simulink model "SF020A_HwAgTrakgServo"  (R2013b)
settings: Solver=FixedStepDiscrete  SolverMode=SingleTasking  StartTime=0.0  StopTime=1  FixedStep=0.002  RelTol=1e-3
undefined symbols (not defined in the file): ARCHGLBPRM_2MILLISEC_SEC_F32, HwAgTrakgServoEnaRate, HwAgTrakgServoExecRate, HwAgTrakgServoMaxRamp, HwAgTrakgServoPidLim, HwAgTrakgServoRampCmpl, SYSGLBPRM_MOTTQCMDHILIM_MOTNWTMTR_F32, SYSGLBPRM_MOTTQCMDLOLIM_MOTNWTMTR_F32
libraries: FixdToFloat x9, FloatToFixd x8, LnrIntrpn x7, NxtrLim x7, Fil x6, simulink x3, NxtrAbslt x2, BilnrIntrpnCmnX x2, NxtrSign x2
(part 2 of 2)

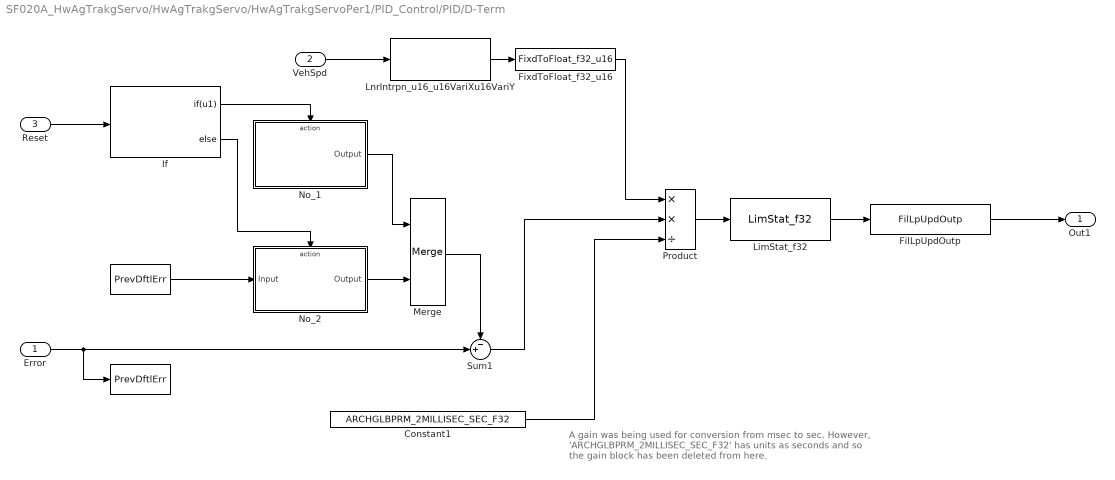
== system SF020A_HwAgTrakgServo/HwAgTrakgServo/HwAgTrakgServoPer1/PID_Control/PID/D-Term ==
  note: A gain was being used for conversion from msec to sec.
      | However, 'ARCHGLBPRM_2MILLISEC_SEC_F32' has units
      | as seconds and so the gain block has been deleted from here.
  Error : Inport
  VehSpd : Inport  RequirementInfo={'linktype_rmi_doors' '0000a533 (/E-STEER Core/SubSystem Specifications/Application Functions/SF020A Position Tracking Servo)' '#SF020A_120' 'true' 'REQ:SF020A_120' '' } %GIDa_d32483ba_765c_4e7c_9854_4c9d7c34dac7  Port=2
  Reset : Inport  Port=3
  "  " : DataStoreWrite  RequirementInfo={'linktype_rmi_doors' '0000a533 (/E-STEER Core/SubSystem Specifications/Application Functions/SF020A Position Tracking Servo)' '#SF020A_120' 'true' 'REQ:SF020A_120' '' } %GIDa_7a2ff437_0271_4ce9_818a_ade8654f46bb  DataStoreName=PrevDftlErr
  " " : DataStoreRead  RequirementInfo={'linktype_rmi_doors' '0000a533 (/E-STEER Core/SubSystem Specifications/Application Functions/SF020A Position Tracking Servo)' '#SF020A_121' 'true' 'REQ:SF020A_121' '' } %GIDa_b646c468_9863_49bd_b902_8e22191691a8  DataStoreName=PrevDftlErr
  Constant1 : Constant  RequirementInfo={'linktype_rmi_doors' '0000a533 (/E-STEER Core/SubSystem Specifications/Application Functions/SF020A Position Tracking Servo)' '#SF020A_120' 'true' 'REQ:SF020A_120' '' } %GIDa_1ecc393f_7cc1_4c4e_8080_3b7a410d844f  Value=ARCHGLBPRM_2MILLISEC_SEC_F32
  FilLpUpdOutp : Fil/FilLpUpdOutp  RequirementInfo="{'linktype_rmi_doors' '0000a533 (/E-STEER Core/SubSystem Specifications/Application Functions/SF020A Position Tracking Servo)' '#SF020A_120' 'true' 'REQ:  SF020A_120' '' } %GIDa_b8410d6a_59fe_4dcb_bcc7_9a13096b2737"  StVar=DftlTermLpFil
      settings: AttributesFormatString=StVar: %<StVar>
  FixdToFloat_f32_u16 : FixdToFloat/FixdToFloat_f32_u16  RequirementInfo="{'linktype_rmi_doors' '0000a533 (/E-STEER Core/SubSystem Specifications/Application Functions/SF020A Position Tracking Servo)' '#SF020A_120' 'true' 'REQ:  SF020A_120' '' } %GIDa_8cac592f_9679_46eb_895c_0d05cfe3ff7b"  Param1=16
  If : If  RequirementInfo={'linktype_rmi_doors' '0000a533 (/E-STEER Core/SubSystem Specifications/Application Functions/SF020A Position Tracking Servo)' '#SF020A_121' 'true' 'REQ:SF020A_121' '' } %GIDa_2482da2c_29e3_486b_be60_b311b38fc278  IfExpression=u1
  LimStat_f32 : NxtrLim/LimStat_f32  RequirementInfo="{'linktype_rmi_doors' '0000a533 (/E-STEER Core/SubSystem Specifications/Application Functions/SF020A Position Tracking Servo)' '#SF020A_120' 'true' 'REQ:  SF020A_120' '' } %GIDa_56604264_d76a_420a_89c8_0243c47d2796"  LoLim=DFTLTERMMIN_MOTNWTMTR_F32  HiLim=DFTLTERMMAX_MOTNWTMTR_F32
      settings: AttributesFormatString=|
      | Low Limit: %<LoLim>
      | High Limit:%<HiLim>
  LnrIntrpn_u16_u16VariXu16VariY : LnrIntrpn/LnrIntrpn_u16_u16VariXu16VariY  RequirementInfo="{'linktype_rmi_doors' '0000a533 (/E-STEER Core/SubSystem Specifications/Application Functions/SF020A Position Tracking Servo)' '#SF020A_120' 'true' 'REQ:  SF020A_120' '' ; 'linktype_rmi_doors' '0000a533 (/E-STEER Core/SubSystem Specifications/Application Functions/SF020A Position Tracking Servo)' '#SF020A_121' 'true' 'REQ:  SF020A_121' '' } %GIDa_2e6fa66c_d77a_4943_945e_e25c3e6f5b3b"  XTbl=HwAgTrakgServoVehSpdBasd  YTbl=HwAgTrakgServoDftlGainY
      settings: AttributesFormatString=Lnr ( u16VariX , u16VariY )
  Merge : Merge  RequirementInfo={'linktype_rmi_doors' '0000a533 (/E-STEER Core/SubSystem Specifications/Application Functions/SF020A Position Tracking Servo)' '#SF020A_121' 'true' 'REQ:SF020A_121' '' } %GIDa_db000ce9_21e4_46f6_81ad_8c041347f9e5
  No_1 : Subsystem  RequirementInfo={'linktype_rmi_doors' '0000a533 (/E-STEER Core/SubSystem Specifications/Application Functions/SF020A Position Tracking Servo)' '#SF020A_121' 'true' 'REQ:SF020A_121' '' } %GIDa_913a8a21_a22e_47bf_9e83_df1d046cce8d  TreatAsAtomicUnit=on
  No_2 : Subsystem  RequirementInfo={'linktype_rmi_doors' '0000a533 (/E-STEER Core/SubSystem Specifications/Application Functions/SF020A Position Tracking Servo)' '#SF020A_121' 'true' 'REQ:SF020A_121' '' } %GIDa_9df1ffb9_cc87_486c_93e5_5eb2c3c347a7  TreatAsAtomicUnit=on
  Product : Product  RequirementInfo={'linktype_rmi_doors' '0000a533 (/E-STEER Core/SubSystem Specifications/Application Functions/SF020A Position Tracking Servo)' '#SF020A_120' 'true' 'REQ:SF020A_120' '' } %GIDa_10f02c07_eab9_451a_9a4c_01a4745aac1a  Inputs=**/  RndMeth=Zero
  Sum1 : Sum  RequirementInfo={'linktype_rmi_doors' '0000a533 (/E-STEER Core/SubSystem Specifications/Application Functions/SF020A Position Tracking Servo)' '#SF020A_120' 'true' 'REQ:SF020A_120' '' } %GIDa_669423b0_1be1_4fee_ba39_26e793d23548  Inputs=-+|
  Out1 : Outport
  wires:
  Sum1/1 -> Product/2
  Product/1 -> LimStat_f32/1
  LimStat_f32/1 -> FilLpUpdOutp/1
  FilLpUpdOutp/1 -> Out1/1
  Constant1/1 -> Product/3
  VehSpd/1 -> LnrIntrpn_u16_u16VariXu16VariY/1
  LnrIntrpn_u16_u16VariXu16VariY/1 -> FixdToFloat_f32_u16/1
  FixdToFloat_f32_u16/1 -> Product/1
  If/1 -> No_1/Action
  No_1/1(Output) -> Merge/1
  Merge/1 -> Sum1/1
  If/2 -> No_2/Action
  No_2/1(Output) -> Merge/2
  Reset/1 -> If/1
  Error/1 -> "  "/1, Sum1/2
  " "/1 -> No_2/1(Input)

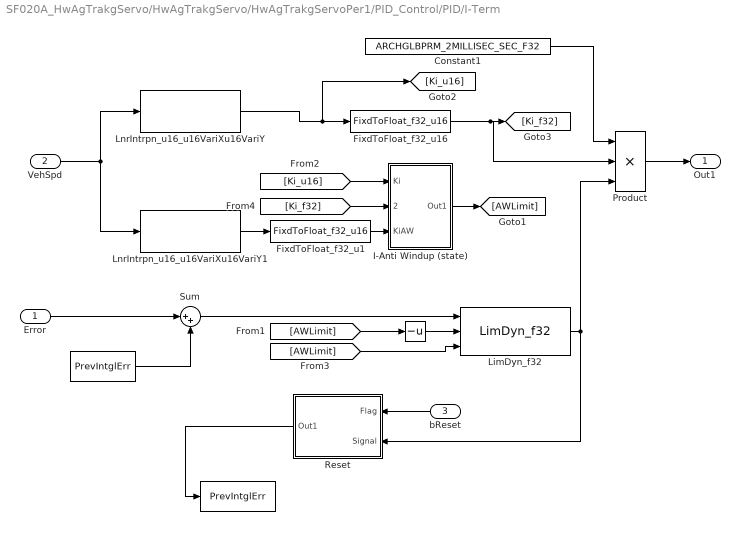
== system SF020A_HwAgTrakgServo/HwAgTrakgServo/HwAgTrakgServoPer1/PID_Control/PID/I-Term ==
  Error : Inport
  VehSpd : Inport  Port=2
  bReset : Inport  RequirementInfo={'linktype_rmi_doors' '0000a533 (/E-STEER Core/SubSystem Specifications/Application Functions/SF020A Position Tracking Servo)' '#SF020A_118' 'true' 'REQ:SF020A_118' '' } %GIDa_42cbd73d_d21d_4d14_befd_3c7d0ce0296a  Port=3
  " " : UnaryMinus  RequirementInfo={'linktype_rmi_doors' '0000a533 (/E-STEER Core/SubSystem Specifications/Application Functions/SF020A Position Tracking Servo)' '#SF020A_117' 'true' 'REQ:SF020A_117' '' } %GIDa_89f9ccfb_a876_46d8_9437_2574eb60ea80
  "    " : DataStoreRead  RequirementInfo={'linktype_rmi_doors' '0000a533 (/E-STEER Core/SubSystem Specifications/Application Functions/SF020A Position Tracking Servo)' '#SF020A_116' 'true' 'REQ:SF020A_116' '' } %GIDa_32ef5a5c_1147_48c1_a2b1_c99166101285  DataStoreName=PrevIntglErr
  "                      " : DataStoreWrite  RequirementInfo={'linktype_rmi_doors' '0000a533 (/E-STEER Core/SubSystem Specifications/Application Functions/SF020A Position Tracking Servo)' '#SF020A_118' 'true' 'REQ:SF020A_118' '' } %GIDa_fefcbefd_ce0f_4bfb_82a6_01cc1f5b96d1  DataStoreName=PrevIntglErr
  Constant1 : Constant  RequirementInfo={'linktype_rmi_doors' '0000a533 (/E-STEER Core/SubSystem Specifications/Application Functions/SF020A Position Tracking Servo)' '#SF020A_116' 'true' 'REQ:SF020A_116' '' } %GIDa_c7ba7a95_a44d_4b4f_9268_9abd4fc5ade3  Value=ARCHGLBPRM_2MILLISEC_SEC_F32
  FixdToFloat_f32_u1 : FixdToFloat/FixdToFloat_f32_u16  RequirementInfo="{'linktype_rmi_doors' '0000a533 (/E-STEER Core/SubSystem Specifications/Application Functions/SF020A Position Tracking Servo)' '#SF020A_117' 'true' 'REQ:  SF020A_117' '' } %GIDa_9607823e_5536_4c8d_af66_ea7d7950732e"  Param1=6
  FixdToFloat_f32_u16 : FixdToFloat/FixdToFloat_f32_u16  RequirementInfo="{'linktype_rmi_doors' '0000a533 (/E-STEER Core/SubSystem Specifications/Application Functions/SF020A Position Tracking Servo)' '#SF020A_116' 'true' 'REQ:  SF020A_116' '' } %GIDa_4b7f174a_bb9c_4a9b_b796_dd3c07e76341"  Param1=14
  I-Anti Windup (state) : Subsystem  RequirementInfo={'linktype_rmi_doors' '0000a533 (/E-STEER Core/SubSystem Specifications/Application Functions/SF020A Position Tracking Servo)' '#SF020A_117' 'true' 'REQ:SF020A_117' '' } %GIDa_dca58060_bf1a_4dc6_9992_f6ed7f7bbb23
  LimDyn_f32 : NxtrLim/LimDyn_f32  RequirementInfo="{'linktype_rmi_doors' '0000a533 (/E-STEER Core/SubSystem Specifications/Application Functions/SF020A Position Tracking Servo)' '#SF020A_116' 'true' 'REQ:  SF020A_116' '' ; 'linktype_rmi_doors' '0000a533 (/E-STEER Core/SubSystem Specifications/Application Functions/SF020A Position Tracking Servo)' '#SF020A_117' 'true' 'REQ:  SF020A_117' '' } %GIDa_ca105d8f_6163_4cbf_9b3e_ae7ab7ff5ed0"
  LnrIntrpn_u16_u16VariXu16VariY : LnrIntrpn/LnrIntrpn_u16_u16VariXu16VariY  RequirementInfo="{'linktype_rmi_doors' '0000a533 (/E-STEER Core/SubSystem Specifications/Application Functions/SF020A Position Tracking Servo)' '#SF020A_116' 'true' 'REQ:  SF020A_116' '' } %GIDa_3733ef7e_4703_4a46_85f1_fe68a759de0a"  XTbl=HwAgTrakgServoVehSpdBasd  YTbl=HwAgTrakgServoIntglGainY
      settings: AttributesFormatString=Lnr ( u16VariX , u16VariY )
  LnrIntrpn_u16_u16VariXu16VariY1 : LnrIntrpn/LnrIntrpn_u16_u16VariXu16VariY  RequirementInfo="{'linktype_rmi_doors' '0000a533 (/E-STEER Core/SubSystem Specifications/Application Functions/SF020A Position Tracking Servo)' '#SF020A_117' 'true' 'REQ:  SF020A_117' '' } %GIDa_6db552f0_5080_4156_8304_6d32458d9335"  XTbl=HwAgTrakgServoVehSpdBasd  YTbl=HwAgTrakgServoIntglTermAntiWdupLimY
      settings: AttributesFormatString=Lnr ( u16VariX , u16VariY )
  Product : Product  RequirementInfo={'linktype_rmi_doors' '0000a533 (/E-STEER Core/SubSystem Specifications/Application Functions/SF020A Position Tracking Servo)' '#SF020A_116' 'true' 'REQ:SF020A_116' '' } %GIDa_56caf3e8_1c10_495f_ad5a_8190ceb7a18e  Inputs=3  RndMeth=Zero
  Reset : Subsystem  RequirementInfo={'linktype_rmi_doors' '0000a533 (/E-STEER Core/SubSystem Specifications/Application Functions/SF020A Position Tracking Servo)' '#SF020A_118' 'true' 'REQ:SF020A_118' '' } %GIDa_957d8062_cb68_42ad_8831_ed3e1a9ec1f4
  Sum : Sum  RequirementInfo={'linktype_rmi_doors' '0000a533 (/E-STEER Core/SubSystem Specifications/Application Functions/SF020A Position Tracking Servo)' '#SF020A_116' 'true' 'REQ:SF020A_116' '' } %GIDa_d408cf93_9f3d_4841_b3d3_4e2af76f9edd  Inputs=|++
  Out1 : Outport
  wires:
  I-Anti Windup (state)/1(Out1) -> [AWLimit]
  Sum/1 -> LimDyn_f32/1
  Error/1 -> Sum/1
  [AWLimit] -> LimDyn_f32/3
  [AWLimit] -> " "/1
  " "/1 -> LimDyn_f32/2
  LimDyn_f32/1 -> Reset/2(Signal), Product/3
  Product/1 -> Out1/1
  Constant1/1 -> Product/1
  Reset/1(Out1) -> "                      "/1
  bReset/1 -> Reset/1(Flag)
  LnrIntrpn_u16_u16VariXu16VariY/1 -> [Ki_u16], FixdToFloat_f32_u16/1
  FixdToFloat_f32_u16/1 -> [Ki_f32], Product/2
  VehSpd/1 -> LnrIntrpn_u16_u16VariXu16VariY1/1, LnrIntrpn_u16_u16VariXu16VariY/1
  LnrIntrpn_u16_u16VariXu16VariY1/1 -> FixdToFloat_f32_u1/1
  FixdToFloat_f32_u1/1 -> I-Anti Windup (state)/3(KiAW)
  "    "/1 -> Sum/2
  [Ki_f32] -> I-Anti Windup (state)/2(Ki_f32)
  [Ki_u16] -> I-Anti Windup (state)/1(Ki)

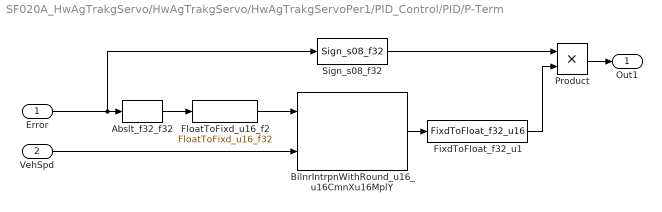
== system SF020A_HwAgTrakgServo/HwAgTrakgServo/HwAgTrakgServoPer1/PID_Control/PID/P-Term ==
  Error : Inport
  VehSpd : Inport  Port=2
  Abslt_f32_f32 : NxtrAbslt/Abslt_f32_f32  RequirementInfo="{'linktype_rmi_doors' '0000a533 (/E-STEER Core/SubSystem Specifications/Application Functions/SF020A Position Tracking Servo)' '#SF020A_112' 'true' 'REQ:  SF020A_112' '' } %GIDa_19b36650_53a9_40a5_a2c3_3e180a66e833"  SFunctionSpec=single y1 = Abslt_f32_f32(single u1)
      settings: AttributesFormatString=%<Name>
  BilnrIntrpnWithRound_u16_u16CmnXu16MplY : BilnrIntrpnCmnX/BilnrIntrpnWithRound_u16_u16CmnXu16MplY  RequirementInfo="{'linktype_rmi_doors' '0000a533 (/E-STEER Core/SubSystem Specifications/Application Functions/SF020A Position Tracking Servo)' '#SF020A_112' 'true' 'REQ:  SF020A_112' '' } %GIDa_31e47da8_032d_42f7_b4f4_30bc796728ea"  XTbl=HwAgTrakgServoPropGainX  MplYTbl=HwAgTrakgServoPropGainY  BilnrSelnTbl=HwAgTrakgServoVehSpdBasd
      settings: AttributesFormatString=Bilnr ( u16CmnX , u16MplY )
  FixdToFloat_f32_u1 : FixdToFloat/FixdToFloat_f32_u16  RequirementInfo="{'linktype_rmi_doors' '0000a533 (/E-STEER Core/SubSystem Specifications/Application Functions/SF020A Position Tracking Servo)' '#SF020A_112' 'true' 'REQ:  SF020A_112' '' } %GIDa_bbd8601d_9849_428a_aee0_f7dbd445b900"  Param1=6
  FloatToFixd_u16_f2 : FloatToFixd/FloatToFixd_u16_f32  RequirementInfo="{'linktype_rmi_doors' '0000a533 (/E-STEER Core/SubSystem Specifications/Application Functions/SF020A Position Tracking Servo)' '#SF020A_112' 'true' 'REQ:  SF020A_112' '' } %GIDa_3f4e1614_69e3_41e7_a5a8_651d4065b758"  Param1=4
  Product : Product  RequirementInfo={'linktype_rmi_doors' '0000a533 (/E-STEER Core/SubSystem Specifications/Application Functions/SF020A Position Tracking Servo)' '#SF020A_112' 'true' 'REQ:SF020A_112' '' } %GIDa_0461f146_b9cd_4837_ab1e_fbfc8fbdcec8  RndMeth=Zero
  Sign_s08_f32 : NxtrSign/Sign_s08_f32  RequirementInfo="{'linktype_rmi_doors' '0000a533 (/E-STEER Core/SubSystem Specifications/Application Functions/SF020A Position Tracking Servo)' '#SF020A_112' 'true' 'REQ:  SF020A_112' '' } %GIDa_bfd997e9_0cca_4785_a7cd_5d86c8a88cbc"  SFunctionSpec=int8 y1 = Sign_s08_f32(single u1)
  Out1 : Outport
  wires:
  Abslt_f32_f32/1 -> FloatToFixd_u16_f2/1
  FixdToFloat_f32_u1/1 -> Product/2
  Error/1 -> Sign_s08_f32/1, Abslt_f32_f32/1
  Product/1 -> Out1/1
  Sign_s08_f32/1 -> Product/1
  VehSpd/1 -> BilnrIntrpnWithRound_u16_u16CmnXu16MplY/2
  FloatToFixd_u16_f2/1 -> BilnrIntrpnWithRound_u16_u16CmnXu16MplY/1
  BilnrIntrpnWithRound_u16_u16CmnXu16MplY/1 -> FixdToFloat_f32_u1/1

== system SF020A_HwAgTrakgServo/HwAgTrakgServo/HwAgTrakgServoPer1/PID_Control/PID/Reset ==
  Flag : Inport
  Signal : Inport  Port=2
  If : If  RequirementInfo={} %GIDa_9823df34_12f0_430f_beda_15da64defd33  IfExpression=u1
  Merge : Merge
  Send_Signal : Subsystem  RequirementInfo={} %GIDa_b55c34b6_726a_4bd6_bd80_9a3ddcc5c4fc  TreatAsAtomicUnit=on
  Send_Zero : Subsystem  RequirementInfo={} %GIDa_f80fb8fa_8646_4de8_8433_4e18c44a8cc0  TreatAsAtomicUnit=on
  Out1 : Outport
  wires:
  Signal/1 -> Send_Signal/1(Input)
  If/1 -> Send_Zero/Action
  Flag/1 -> If/1
  Send_Zero/1(Output) -> Merge/1
  Merge/1 -> Out1/1
  If/2 -> Send_Signal/Action
  Send_Signal/1(Output) -> Merge/2

== system SF020A_HwAgTrakgServo/HwAgTrakgServo/HwAgTrakgServoPer1/PID_Control/PID/Reset1 ==
  Flag : Inport
  Signal : Inport  Port=2
  If : If  RequirementInfo={} %GIDa_eff16e79_4283_44bd_badf_9e4f43f9c0bd  IfExpression=u1
  Merge : Merge
  Send_Signal : Subsystem  RequirementInfo={} %GIDa_73f60ec3_a0bd_4e60_ba0a_9dcd12611295  TreatAsAtomicUnit=on
  Send_Zero : Subsystem  RequirementInfo={} %GIDa_f86147ff_5456_40c2_9d6b_02485c028dcf  TreatAsAtomicUnit=on
  Out1 : Outport
  wires:
  Signal/1 -> Send_Signal/1(Input)
  If/1 -> Send_Zero/Action
  Flag/1 -> If/1
  Send_Zero/1(Output) -> Merge/1
  Merge/1 -> Out1/1
  If/2 -> Send_Signal/Action
  Send_Signal/1(Output) -> Merge/2

== system SF020A_HwAgTrakgServo/HwAgTrakgServo/HwAgTrakgServoPer1/Transition_Control/Disabling_Mech/CopyRight2 ==

== system SF020A_HwAgTrakgServo/HwAgTrakgServo/HwAgTrakgServoPer1/Transition_Control/Enable_Mech/CopyRight2 ==

== system SF020A_HwAgTrakgServo/HwAgTrakgServo/HwAgTrakgServoPer1/PID_Control/PID/D-Term/No_1 ==
  Action Port : ActionPort  ActionType=then
  Constant2 : Constant  Value=0  OutDataTypeStr=single
  CopyRight2 : Subsystem  Description=|  mask(Copyright Information){none=on}
      | Copyright info block.                                               
      |                                                                     
      | Place copyright information at the top of every subsystem in design.
      mask prompts: none "No parameters"
      mask help: Place copyright information at the top of every subsystem in design.
      mask Display:
      | NxtrConf = 'Nexteer Confidential';
      | 
      | sys = bdroot; %handle for the current model ("system")
      | first = get_param(sys,'Created');
      | if(isempty(first))
      |     first = datestr(now,'yyyy');
      | else
      |     first = first(end-3:end);  %year is last four digits
      | end
      | 
      | last = get_param(sys,'LastModifiedDate');
      | if isempty(last)
      |     last = datestr(now,'yyyy');
      | else
      |     last = last(end-3:end);
      | end
      | 
      | if strcmp(first,last)
      |     fprintf('%s -- Copyright %s Nexteer',NxtrConf,first)
      | else
      |     fprintf('%s -- %s%s- %s Nexteer',NxtrConf,char(169),first,last)
      | end
  Output : Outport  InitialOutput=[0]
  wires:
  Constant2/1 -> Output/1

== system SF020A_HwAgTrakgServo/HwAgTrakgServo/HwAgTrakgServoPer1/PID_Control/PID/D-Term/No_2 ==
  Input : Inport
  Action Port : ActionPort  ActionType=else
  CopyRight2 : Subsystem  Description=|  mask(Copyright Information){none=on}
      | Copyright info block.                                               
      |                                                                     
      | Place copyright information at the top of every subsystem in design.
      mask prompts: none "No parameters"
      mask help: Place copyright information at the top of every subsystem in design.
      mask Display:
      | NxtrConf = 'Nexteer Confidential';
      | 
      | sys = bdroot; %handle for the current model ("system")
      | first = get_param(sys,'Created');
      | if(isempty(first))
      |     first = datestr(now,'yyyy');
      | else
      |     first = first(end-3:end);  %year is last four digits
      | end
      | 
      | last = get_param(sys,'LastModifiedDate');
      | if isempty(last)
      |     last = datestr(now,'yyyy');
      | else
      |     last = last(end-3:end);
      | end
      | 
      | if strcmp(first,last)
      |     fprintf('%s -- Copyright %s Nexteer',NxtrConf,first)
      | else
      |     fprintf('%s -- %s%s- %s Nexteer',NxtrConf,char(169),first,last)
      | end
  Output : Outport  InitialOutput=[0]
  wires:
  Input/1 -> Output/1

== system SF020A_HwAgTrakgServo/HwAgTrakgServo/HwAgTrakgServoPer1/PID_Control/PID/I-Term/I-Anti Windup (state) ==
  Ki : Inport
  Ki_f32 : Inport  Port=2
  KiAW : Inport  Port=3
  If : If  IfExpression=u1 == 0
  Ki=0 : Subsystem  TreatAsAtomicUnit=on
  Ki~=0 : Subsystem  TreatAsAtomicUnit=on
  Merge : Merge
  Out1 : Outport
  wires:
  If/1 -> Ki=0/Action
  If/2 -> Ki~=0/Action
  Ki=0/1(Out1) -> Merge/1
  Ki~=0/1(Out1) -> Merge/2
  Ki/1 -> If/1
  Merge/1 -> Out1/1
  KiAW/1 -> Ki~=0/2(KiAW)
  Ki_f32/1 -> Ki~=0/1(Ki)

== system SF020A_HwAgTrakgServo/HwAgTrakgServo/HwAgTrakgServoPer1/PID_Control/PID/I-Term/Reset ==
  Flag : Inport
  Signal : Inport  Port=2
  If : If  RequirementInfo={} %GIDa_9f6dddb6_da7f_44ce_b372_08d15591f6a9  IfExpression=u1
  Merge : Merge
  Send_Signal : Subsystem  RequirementInfo={} %GIDa_cda83b5e_6fbf_4df5_babd_5f7f9e6e4c79  TreatAsAtomicUnit=on
  Send_Zero : Subsystem  RequirementInfo={} %GIDa_5b51831a_4950_4671_9e3b_80d5386ccfbf  TreatAsAtomicUnit=on
  Out1 : Outport
  wires:
  Signal/1 -> Send_Signal/1(Input)
  If/1 -> Send_Zero/Action
  Flag/1 -> If/1
  Send_Zero/1(Output) -> Merge/1
  If/2 -> Send_Signal/Action
  Send_Signal/1(Output) -> Merge/2
  Merge/1 -> Out1/1

== system SF020A_HwAgTrakgServo/HwAgTrakgServo/HwAgTrakgServoPer1/PID_Control/PID/Reset/Send_Signal ==
  Input : Inport
  Action Port : ActionPort  ActionType=else
  CopyRight2 : Subsystem  Description=|  mask(Copyright Information){none=on}
      | Copyright info block.                                               
      |                                                                     
      | Place copyright information at the top of every subsystem in design.
      mask prompts: none "No parameters"
      mask help: Place copyright information at the top of every subsystem in design.
      mask Display:
      | NxtrConf = 'Nexteer Confidential';
      | 
      | sys = bdroot; %handle for the current model ("system")
      | first = get_param(sys,'Created');
      | if(isempty(first))
      |     first = datestr(now,'yyyy');
      | else
      |     first = first(end-3:end);  %year is last four digits
      | end
      | 
      | last = get_param(sys,'LastModifiedDate');
      | if isempty(last)
      |     last = datestr(now,'yyyy');
      | else
      |     last = last(end-3:end);
      | end
      | 
      | if strcmp(first,last)
      |     fprintf('%s -- Copyright %s Nexteer',NxtrConf,first)
      | else
      |     fprintf('%s -- %s%s- %s Nexteer',NxtrConf,char(169),first,last)
      | end
  Output : Outport  InitialOutput=[0]
  wires:
  Input/1 -> Output/1

== system SF020A_HwAgTrakgServo/HwAgTrakgServo/HwAgTrakgServoPer1/PID_Control/PID/Reset/Send_Zero ==
  Action Port : ActionPort  ActionType=then
  Constant2 : Constant  Value=0  OutDataTypeStr=single
  CopyRight2 : Subsystem  Description=|  mask(Copyright Information){none=on}
      | Copyright info block.                                               
      |                                                                     
      | Place copyright information at the top of every subsystem in design.
      mask prompts: none "No parameters"
      mask help: Place copyright information at the top of every subsystem in design.
      mask Display:
      | NxtrConf = 'Nexteer Confidential';
      | 
      | sys = bdroot; %handle for the current model ("system")
      | first = get_param(sys,'Created');
      | if(isempty(first))
      |     first = datestr(now,'yyyy');
      | else
      |     first = first(end-3:end);  %year is last four digits
      | end
      | 
      | last = get_param(sys,'LastModifiedDate');
      | if isempty(last)
      |     last = datestr(now,'yyyy');
      | else
      |     last = last(end-3:end);
      | end
      | 
      | if strcmp(first,last)
      |     fprintf('%s -- Copyright %s Nexteer',NxtrConf,first)
      | else
      |     fprintf('%s -- %s%s- %s Nexteer',NxtrConf,char(169),first,last)
      | end
  Output : Outport  InitialOutput=[0]
  wires:
  Constant2/1 -> Output/1

== system SF020A_HwAgTrakgServo/HwAgTrakgServo/HwAgTrakgServoPer1/PID_Control/PID/Reset1/Send_Signal ==
  Input : Inport
  Action Port : ActionPort  ActionType=else
  CopyRight2 : Subsystem  Description=|  mask(Copyright Information){none=on}
      | Copyright info block.                                               
      |                                                                     
      | Place copyright information at the top of every subsystem in design.
      mask prompts: none "No parameters"
      mask help: Place copyright information at the top of every subsystem in design.
      mask Display:
      | NxtrConf = 'Nexteer Confidential';
      | 
      | sys = bdroot; %handle for the current model ("system")
      | first = get_param(sys,'Created');
      | if(isempty(first))
      |     first = datestr(now,'yyyy');
      | else
      |     first = first(end-3:end);  %year is last four digits
      | end
      | 
      | last = get_param(sys,'LastModifiedDate');
      | if isempty(last)
      |     last = datestr(now,'yyyy');
      | else
      |     last = last(end-3:end);
      | end
      | 
      | if strcmp(first,last)
      |     fprintf('%s -- Copyright %s Nexteer',NxtrConf,first)
      | else
      |     fprintf('%s -- %s%s- %s Nexteer',NxtrConf,char(169),first,last)
      | end
  Output : Outport  InitialOutput=[0]
  wires:
  Input/1 -> Output/1

== system SF020A_HwAgTrakgServo/HwAgTrakgServo/HwAgTrakgServoPer1/PID_Control/PID/Reset1/Send_Zero ==
  Action Port : ActionPort  ActionType=then
  Constant2 : Constant  Value=0  OutDataTypeStr=single
  CopyRight2 : Subsystem  Description=|  mask(Copyright Information){none=on}
      | Copyright info block.                                               
      |                                                                     
      | Place copyright information at the top of every subsystem in design.
      mask prompts: none "No parameters"
      mask help: Place copyright information at the top of every subsystem in design.
      mask Display:
      | NxtrConf = 'Nexteer Confidential';
      | 
      | sys = bdroot; %handle for the current model ("system")
      | first = get_param(sys,'Created');
      | if(isempty(first))
      |     first = datestr(now,'yyyy');
      | else
      |     first = first(end-3:end);  %year is last four digits
      | end
      | 
      | last = get_param(sys,'LastModifiedDate');
      | if isempty(last)
      |     last = datestr(now,'yyyy');
      | else
      |     last = last(end-3:end);
      | end
      | 
      | if strcmp(first,last)
      |     fprintf('%s -- Copyright %s Nexteer',NxtrConf,first)
      | else
      |     fprintf('%s -- %s%s- %s Nexteer',NxtrConf,char(169),first,last)
      | end
  Output : Outport  InitialOutput=[0]
  wires:
  Constant2/1 -> Output/1

== system SF020A_HwAgTrakgServo/HwAgTrakgServo/HwAgTrakgServoPer1/PID_Control/PID/D-Term/No_1/CopyRight2 ==

== system SF020A_HwAgTrakgServo/HwAgTrakgServo/HwAgTrakgServoPer1/PID_Control/PID/D-Term/No_2/CopyRight2 ==

== system SF020A_HwAgTrakgServo/HwAgTrakgServo/HwAgTrakgServoPer1/PID_Control/PID/I-Term/I-Anti Windup (state)/Ki=0 ==
  Action Port : ActionPort  ActionType=then
  Constant : Constant  Value=0  OutDataTypeStr=single
  Out1 : Outport  InitialOutput=0
  wires:
  Constant/1 -> Out1/1

== system SF020A_HwAgTrakgServo/HwAgTrakgServo/HwAgTrakgServoPer1/PID_Control/PID/I-Term/I-Anti Windup (state)/Ki~=0 ==
  Ki : Inport
  KiAW : Inport  Port=2
  Action Port : ActionPort  ActionType=else
  Constant1 : Constant  Value=HwAgTrakgServoExecRate
  Product1 : Product  Inputs=**/  RndMeth=Zero
  Out1 : Outport
  wires:
  KiAW/1 -> Product1/2
  Ki/1 -> Product1/3
  Constant1/1 -> Product1/1
  Product1/1 -> Out1/1

== system SF020A_HwAgTrakgServo/HwAgTrakgServo/HwAgTrakgServoPer1/PID_Control/PID/I-Term/Reset/Send_Signal ==
  Input : Inport
  Action Port : ActionPort  ActionType=else
  CopyRight2 : Subsystem  Description=|  mask(Copyright Information){none=on}
      | Copyright info block.                                               
      |                                                                     
      | Place copyright information at the top of every subsystem in design.
      mask prompts: none "No parameters"
      mask help: Place copyright information at the top of every subsystem in design.
      mask Display:
      | NxtrConf = 'Nexteer Confidential';
      | 
      | sys = bdroot; %handle for the current model ("system")
      | first = get_param(sys,'Created');
      | if(isempty(first))
      |     first = datestr(now,'yyyy');
      | else
      |     first = first(end-3:end);  %year is last four digits
      | end
      | 
      | last = get_param(sys,'LastModifiedDate');
      | if isempty(last)
      |     last = datestr(now,'yyyy');
      | else
      |     last = last(end-3:end);
      | end
      | 
      | if strcmp(first,last)
      |     fprintf('%s -- Copyright %s Nexteer',NxtrConf,first)
      | else
      |     fprintf('%s -- %s%s- %s Nexteer',NxtrConf,char(169),first,last)
      | end
  Output : Outport  InitialOutput=[0]
  wires:
  Input/1 -> Output/1

== system SF020A_HwAgTrakgServo/HwAgTrakgServo/HwAgTrakgServoPer1/PID_Control/PID/I-Term/Reset/Send_Zero ==
  Action Port : ActionPort  ActionType=then
  Constant2 : Constant  Value=0  OutDataTypeStr=single
  CopyRight2 : Subsystem  Description=|  mask(Copyright Information){none=on}
      | Copyright info block.                                               
      |                                                                     
      | Place copyright information at the top of every subsystem in design.
      mask prompts: none "No parameters"
      mask help: Place copyright information at the top of every subsystem in design.
      mask Display:
      | NxtrConf = 'Nexteer Confidential';
      | 
      | sys = bdroot; %handle for the current model ("system")
      | first = get_param(sys,'Created');
      | if(isempty(first))
      |     first = datestr(now,'yyyy');
      | else
      |     first = first(end-3:end);  %year is last four digits
      | end
      | 
      | last = get_param(sys,'LastModifiedDate');
      | if isempty(last)
      |     last = datestr(now,'yyyy');
      | else
      |     last = last(end-3:end);
      | end
      | 
      | if strcmp(first,last)
      |     fprintf('%s -- Copyright %s Nexteer',NxtrConf,first)
      | else
      |     fprintf('%s -- %s%s- %s Nexteer',NxtrConf,char(169),first,last)
      | end
  Output : Outport  InitialOutput=[0]
  wires:
  Constant2/1 -> Output/1

== system SF020A_HwAgTrakgServo/HwAgTrakgServo/HwAgTrakgServoPer1/PID_Control/PID/Reset/Send_Signal/CopyRight2 ==

== system SF020A_HwAgTrakgServo/HwAgTrakgServo/HwAgTrakgServoPer1/PID_Control/PID/Reset/Send_Zero/CopyRight2 ==

== system SF020A_HwAgTrakgServo/HwAgTrakgServo/HwAgTrakgServoPer1/PID_Control/PID/Reset1/Send_Signal/CopyRight2 ==

== system SF020A_HwAgTrakgServo/HwAgTrakgServo/HwAgTrakgServoPer1/PID_Control/PID/Reset1/Send_Zero/CopyRight2 ==

== system SF020A_HwAgTrakgServo/HwAgTrakgServo/HwAgTrakgServoPer1/PID_Control/PID/I-Term/Reset/Send_Signal/CopyRight2 ==

== system SF020A_HwAgTrakgServo/HwAgTrakgServo/HwAgTrakgServoPer1/PID_Control/PID/I-Term/Reset/Send_Zero/CopyRight2 ==
